simulink model "sampleModel2062_4"  (R2023a)
settings: Solver=VariableStepAuto  StartTime=0.0  StopTime=10.0  RelTol=1e-3
libraries: simulink x2
settings Model: Creator=user1  LastModifiedBy=user1

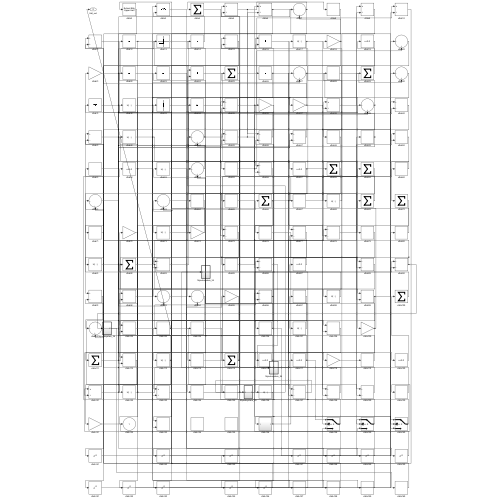
[thumbnail: Simulink's stored preview of the top-level diagram]
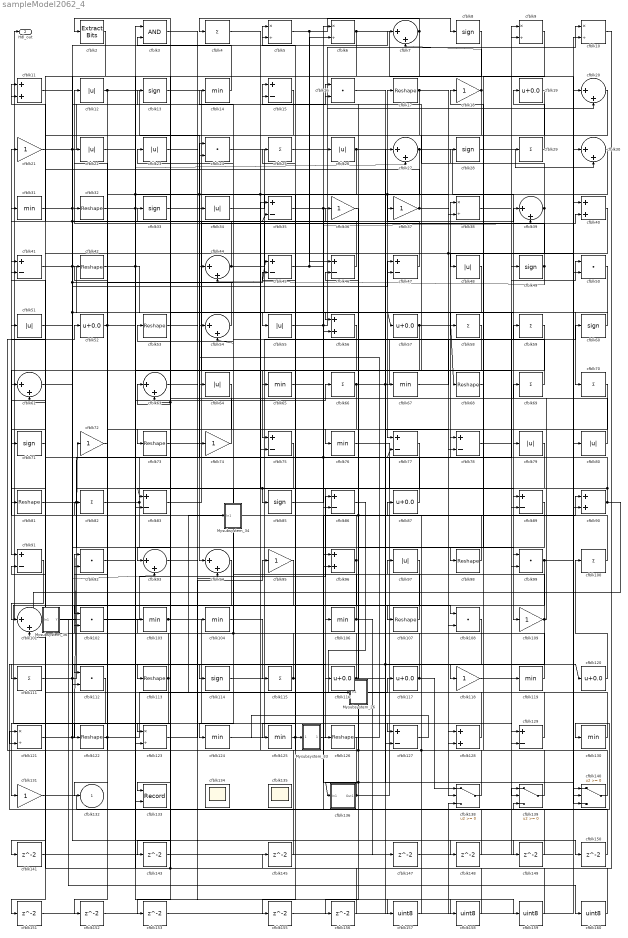
== system sampleModel2062_4 ==
  Mysubsystem_26 : Subsystem  TreatAsAtomicUnit=on  RTWFcnName=Mysubsystem_26
      settings: RTWFcnNameOpts=User specified  RTWFileNameOpts=Use function name
  Mysubsystem_33 : Subsystem  TreatAsAtomicUnit=on  RTWFcnName=Mysubsystem_33
      settings: RTWFcnNameOpts=User specified  RTWFileNameOpts=Use function name
  Mysubsystem_34 : Subsystem  TreatAsAtomicUnit=on  RTWFcnName=Mysubsystem_34
      settings: RTWFcnNameOpts=User specified  RTWFileNameOpts=Use function name
  Mysubsystem_36 : Subsystem  TreatAsAtomicUnit=on  RTWFcnName=Mysubsystem_36
      settings: RTWFcnNameOpts=User specified  RTWFileNameOpts=Use function name
  cfblk{5..6,9..10,38,121,123} (7 alike) : Product  Inputs=*/  OutDataTypeStr=uint8  RndMeth=Zero  SaturateOnIntegerOverflow=on
  cfblk{4,25,29,58..59,66,69..70,82,100,111,115} (12 alike) : Sum  Inputs=+  OutDataTypeStr=uint8
  cfblk{7,20,27,30,39,44,54,61,63,93..94,101} (12 alike) : Sum  Inputs=|++  OutDataTypeStr=uint8
  cfblk{16,24,50,92,99,102,108,112} (8 alike) : DotProduct  OutDataTypeStr=uint8
  cfblk{14,31,65,67,76,103..104,106,119,124..125,130} (12 alike) : MinMax  OutDataTypeStr=uint8
  cfblk{17,32,42,53,68,73,81,98,107,113,122,126} (12 alike) : Reshape
  cfblk{18,21,36..37,72,74,95,109,118,131} (10 alike) : Gain  OutDataTypeStr=uint8
  cfblk{11,40,56,90,96,128} (6 alike) : Sum  OutDataTypeStr=uint8
  cfblk{8,13,28,33,49,60,71,85,114} (9 alike) : Signum
  cfblk{19,52,57,87,116..117,120} (7 alike) : Bias  Bias=0.0  SaturateOnIntegerOverflow=off
  cfblk{12,22..23,26,34,48,51,55,64,79..80,97} (12 alike) : Abs  OutDataTypeStr=uint8  SaturateOnIntegerOverflow=off
  cfblk{15,35,41,45..47,75,77..78,83,86,89,91,127,129} (15 alike) : Sum  Inputs=+-  OutDataTypeStr=uint8
  cfblk133 : Record  FileSettingsInternal="{\"entries\":[{\"content\":{\"excelSettings\":{\"content\":{},\"type\":\"Streamout.ExcelSettings\"}},\"type\":\"Streamout.FileSettingStorage\",\"uuid\":\"\"}],\"packageUris\":[\"http:\\/\\/schema.mathworks.com\\/mf0\\/streamout_blocks\\/R2020a\"],\"version\":\"1.0\"}"  Layout=[1 1]  SignalsInternal="{\"entries\":[{\"content\":{\"signals\":[{\"content\":{\"blockPath\":[],\"dimensions\":[1],\"domain\":\"\",\"lineColor\":\"#a2142f\",\"plots\":[1],\"port\":1,\"signalID\":60930,\"signalName\":\"cfblk97\"},\"type\":\"RecordBlkView.Signal\",\"uuid\":\"\"},{\"content\":{\"blockPath\":[],\"dimensions\":[1],\"domain\":\"\",\"lineColor\":\"#139fff\",\"plots\":[1],\"port\":2,\"signalID\":60933,\"signalName\":\"cfblk30\"},\"type\":\"RecordBlkView.Signal\",\"uuid\":\"\"}]},\"type\":\"RecordBlkView.InputSignals\",\"uuid\":\"\"}],\"packageUris\":[\"http:\\/\\/schema.mathworks.com\\/mf0\\/streamout_blocks\\/R2020a\"],\"version\":\"1.0\"}"  VisualizationBindings="{\"xyplotplugin\":{\"info\":[{\"series\":[{\"bindingParametersList\":[{\"parameter\":\"X-Axis\",\"signalID\":60930,\"signalName\":\"cfblk97\"},{\"parameter\":\"Y-Axis\",\"signalID\":60933,\"signalName\":\"cfblk30\"}],\"seriesID\":23448}],\"subplotID\":1}]}}"  CompatibilityTag=XY  st=-1
  cfblk134 : Scope
      settings: Floating=on
  cfblk135 : Scope
      settings: Floating=on
  cfblk136 : Subsystem
      settings: LibrarySourceBlock=|
      | hdlsllib/Ports &
      | Subsystems/Subsystem
  cfblk138 : Switch  OutDataTypeStr=uint8  SaturateOnIntegerOverflow=off  InputSameDT=off
  cfblk139 : Switch  OutDataTypeStr=uint8  SaturateOnIntegerOverflow=off  InputSameDT=off
  cfblk140 : Switch  OutDataTypeStr=uint8  SaturateOnIntegerOverflow=off  InputSameDT=off
  cfblk{141,143,145,147..153,155..156} (12 alike) : Delay  SampleTime=1
  cfblk{157..160} (4 alike) : DataTypeConversion  OutDataTypeStr=uint8  SaturateOnIntegerOverflow=off  RndMeth=Floor
  cfblk2 : simulink/Logic and Bit Operations/Extract Bits  bitsToExtract=Upper half  numBits=8  bitIdxRange=[0 7]  outScalingMode=Preserve fixed-point scaling
      settings: LibrarySourceBlock=|
      | hdlsllib/Logic and Bit
      | Operations/Extract Bits
  cfblk3 : Logic  AllPortsSameDT=off  OutDataTypeStr=boolean
  cfblk132 : Outport  OutDataTypeStr=uint8  VectorParamsAs1DForOutWhenUnconnected=off
  Hdl_out : Outport  Port=2  OutDataTypeStr=uint8
  wires:
  cfblk30/1 -> cfblk34/1, cfblk133/2, cfblk75/2, cfblk77/1
  cfblk136/1(Out1) -> cfblk38/1, cfblk42/1
  cfblk29/1 -> cfblk19/1
  cfblk13/1 -> cfblk55/1
  cfblk47/1 -> cfblk17/1
  cfblk69/1 -> cfblk23/1
  cfblk56/1 -> cfblk91/1
  cfblk32/1 -> cfblk27/2, cfblk158/1
  cfblk120/1 -> cfblk100/1
  cfblk19/1 -> cfblk93/1, cfblk63/2
  cfblk12/1 -> cfblk94/1, cfblk132/1
  cfblk101/1 -> cfblk107/1
  cfblk27/1 -> cfblk109/1, cfblk155/1
  cfblk14/1 -> cfblk2/1
  cfblk90/1 -> Mysubsystem_36/1(In1), cfblk85/1, cfblk83/1, cfblk41/1
  cfblk71/1 -> cfblk127/1
  cfblk81/1 -> cfblk89/1, cfblk138/2
  cfblk121/1 -> cfblk35/2, cfblk7/1, cfblk45/1, cfblk72/1
  cfblk114/1 -> cfblk9/1
  cfblk126/1 -> cfblk52/1
  cfblk16/1 -> cfblk118/1
  cfblk98/1 -> cfblk21/1
  cfblk140/1 -> cfblk87/1, cfblk36/1
  cfblk109/1 -> cfblk14/1, cfblk69/1, cfblk123/2
  cfblk79/1 -> cfblk127/2
  cfblk52/1 -> cfblk122/1, cfblk159/1
  cfblk49/1 -> cfblk12/1, cfblk44/2
  cfblk51/1 -> cfblk57/1, cfblk47/1
  cfblk131/1 -> cfblk130/1
  cfblk41/1 -> cfblk139/2, cfblk93/2
  cfblk55/1 -> cfblk10/1, cfblk39/2
  cfblk96/1 -> cfblk32/1, cfblk114/1
  cfblk111/1 -> cfblk24/1, cfblk47/2
  cfblk50/1 -> cfblk70/1
  cfblk122/1 -> cfblk117/1, cfblk92/2
  cfblk77/1 -> cfblk126/1
  cfblk112/1 -> cfblk131/1
  cfblk42/1 -> cfblk56/1, cfblk65/1
  cfblk38/1 -> cfblk9/2
  cfblk130/1 -> cfblk61/1
  cfblk124/1 -> cfblk60/1
  cfblk5/1 -> cfblk8/1, cfblk46/1
  cfblk21/1 -> cfblk13/1, cfblk96/2
  cfblk57/1 -> cfblk68/1, cfblk75/1
  cfblk64/1 -> cfblk73/1
  cfblk102/1 -> cfblk86/1
  cfblk58/1 -> cfblk136/1(In1), cfblk156/1
  cfblk66/1 -> cfblk10/2, cfblk78/2, cfblk86/2
  cfblk125/1 -> cfblk15/1, cfblk90/1
  cfblk24/1 -> cfblk79/1
  cfblk91/1 -> cfblk101/1
  cfblk8/1 -> cfblk113/1
  cfblk104/1 -> cfblk115/1
  cfblk113/1 -> cfblk102/2, cfblk151/1
  cfblk73/1 -> cfblk40/2
  cfblk89/1 -> cfblk106/1
  cfblk15/1 -> cfblk101/2
  cfblk83/1 -> cfblk39/1
  cfblk80/1 -> cfblk31/1
  cfblk18/1 -> cfblk67/1, cfblk7/2
  cfblk76/1 -> cfblk119/1
  cfblk37/1 -> cfblk128/1, cfblk11/2
  cfblk103/1 -> cfblk128/2, Hdl_out/1
  cfblk74/1 -> cfblk33/1
  cfblk100/1 -> cfblk5/1, cfblk46/2
  cfblk68/1 -> cfblk18/1
  cfblk53/1 -> cfblk94/2
  cfblk92/1 -> cfblk66/1
  cfblk138/1 -> cfblk16/1, cfblk45/2
  cfblk106/1 -> cfblk44/1, cfblk147/1
  cfblk129/1 -> cfblk5/2
  cfblk118/1 -> cfblk129/1
  cfblk97/1 -> cfblk133/1
  cfblk35/1 -> cfblk20/2, cfblk140/2
  cfblk78/1 -> cfblk50/1
  cfblk119/1 -> cfblk103/1
  cfblk39/1 -> cfblk71/1, cfblk15/2
  cfblk4/1 -> cfblk89/2
  cfblk34/1 -> cfblk37/1
  cfblk54/1 -> cfblk22/1
  cfblk28/1 -> cfblk30/2
  cfblk59/1 -> cfblk64/1
  cfblk116/1 -> cfblk92/1, cfblk78/1
  cfblk26/1 -> cfblk120/1, cfblk140/3, cfblk112/1
  cfblk67/1 -> cfblk59/1
  cfblk46/1 -> cfblk24/2
  cfblk6/1 -> cfblk140/1, cfblk83/2
  cfblk20/1 -> cfblk98/1
  cfblk115/1 -> cfblk25/1, cfblk91/2
  cfblk75/1 -> cfblk124/1
  cfblk7/1 -> cfblk4/1, cfblk112/2
  cfblk61/1 -> cfblk99/1
  cfblk99/1 -> cfblk80/1, cfblk153/1
  cfblk139/1 -> cfblk28/1
  cfblk25/1 -> cfblk26/1
  cfblk87/1 -> cfblk61/2
  cfblk123/1 -> cfblk95/1
  cfblk36/1 -> cfblk76/1
  cfblk33/1 -> cfblk99/2
  cfblk60/1 -> cfblk58/1
  cfblk9/1 -> cfblk48/1
  cfblk82/1 -> cfblk104/1, cfblk49/1
  cfblk72/1 -> cfblk102/1
  cfblk108/1 -> cfblk121/2
  cfblk44/1 -> cfblk29/1, cfblk11/1
  cfblk22/1 -> cfblk38/2, cfblk108/2
  cfblk65/1 -> cfblk108/1
  cfblk40/1 -> cfblk125/1
  cfblk107/1 -> cfblk53/1
  cfblk23/1 -> cfblk74/1
  cfblk17/1 -> cfblk129/2, cfblk50/2, cfblk81/1
  cfblk117/1 -> cfblk54/2, cfblk82/1, cfblk138/1
  cfblk94/1 -> cfblk123/1
  cfblk45/1 -> cfblk56/2, cfblk6/2
  cfblk2/1 -> cfblk111/1
  cfblk31/1 -> cfblk116/1, cfblk16/2
  cfblk85/1 -> cfblk6/1, cfblk77/2
  cfblk95/1 -> cfblk141/1
  cfblk141/1 -> cfblk40/1
  cfblk48/1 -> cfblk143/1
  cfblk143/1 -> cfblk139/1
  cfblk10/1 -> cfblk145/1
  cfblk145/1 -> cfblk35/1
  cfblk147/1 -> cfblk30/1
  cfblk93/1 -> cfblk148/1
  cfblk148/1 -> cfblk96/1
  cfblk63/1 -> cfblk149/1
  cfblk149/1 -> cfblk139/3
  cfblk11/1 -> cfblk150/1
  cfblk150/1 -> cfblk121/1
  cfblk151/1 -> cfblk27/1
  cfblk70/1 -> cfblk152/1
  cfblk152/1 -> cfblk20/1
  cfblk153/1 -> cfblk138/3
  cfblk155/1 -> cfblk90/2
  cfblk156/1 -> cfblk41/2
  cfblk3/1 -> cfblk157/1
  cfblk157/1 -> cfblk97/1
  cfblk158/1 -> cfblk3/1
  cfblk159/1 -> cfblk3/2
  cfblk160/1 -> cfblk63/1, cfblk51/1
  cfblk86/1 -> Mysubsystem_26/1(In1)
  cfblk127/1 -> Mysubsystem_33/1(In1)
  Mysubsystem_33/1(Out1) -> cfblk54/1
  cfblk128/1 -> Mysubsystem_34/1(In1)
  Mysubsystem_36/1(Y) -> cfblk160/1

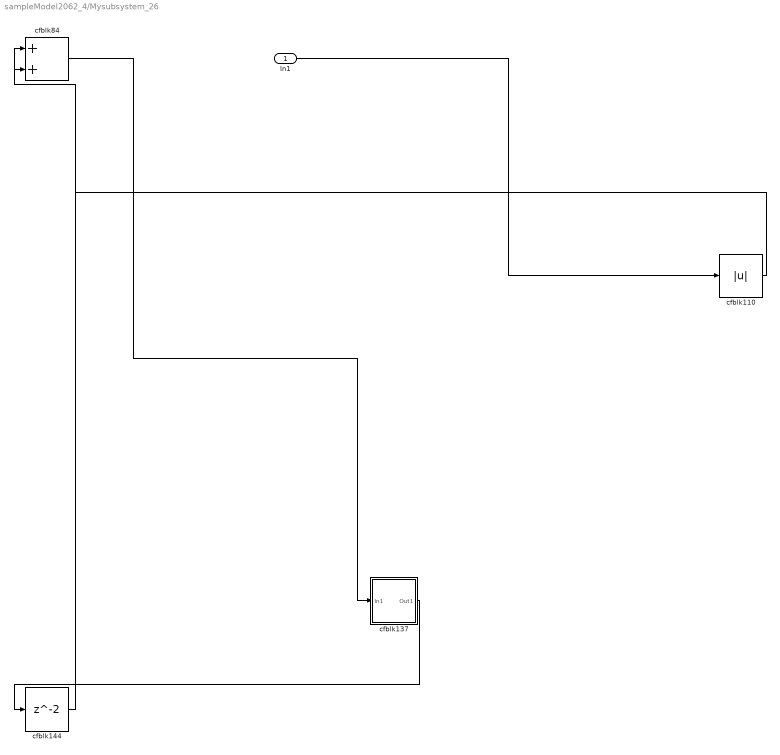
== system sampleModel2062_4/Mysubsystem_26 ==
  In1 : Inport
  cfblk110 : Abs  SaturateOnIntegerOverflow=off
  cfblk137 : Subsystem
      settings: LibrarySourceBlock=|
      | hdlsllib/Ports &
      | Subsystems/Subsystem
  cfblk144 : Delay  SampleTime=1
  cfblk84 : Sum
  wires:
  cfblk110/1 -> cfblk84/1
  cfblk84/1 -> cfblk137/1(In1)
  cfblk137/1(Out1) -> cfblk144/1
  In1/1 -> cfblk110/1
  cfblk144/1 -> cfblk84/2

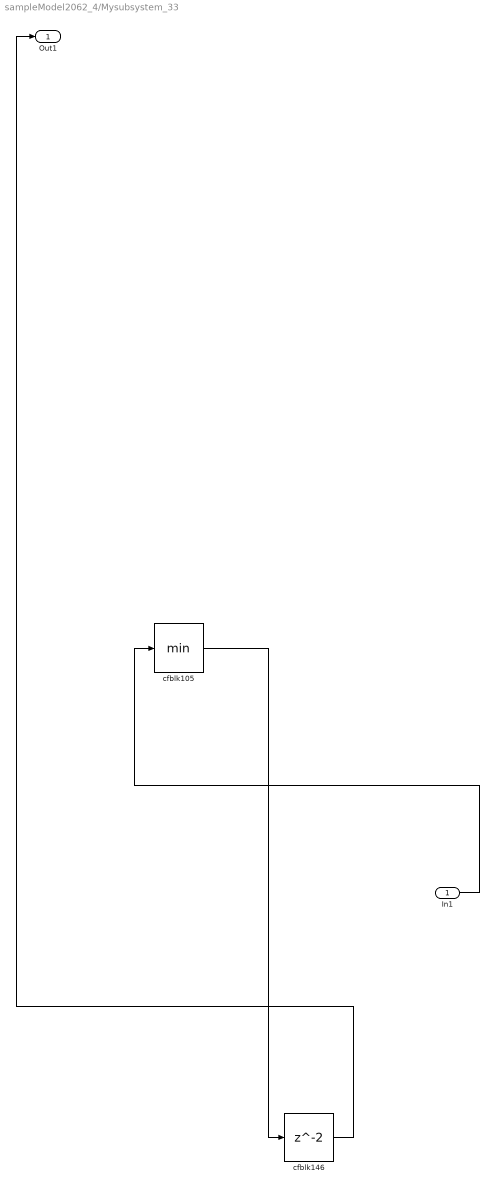
== system sampleModel2062_4/Mysubsystem_33 ==
  In1 : Inport
  cfblk105 : MinMax
  cfblk146 : Delay  SampleTime=1
  Out1 : Outport
  wires:
  cfblk105/1 -> cfblk146/1
  In1/1 -> cfblk105/1
  cfblk146/1 -> Out1/1

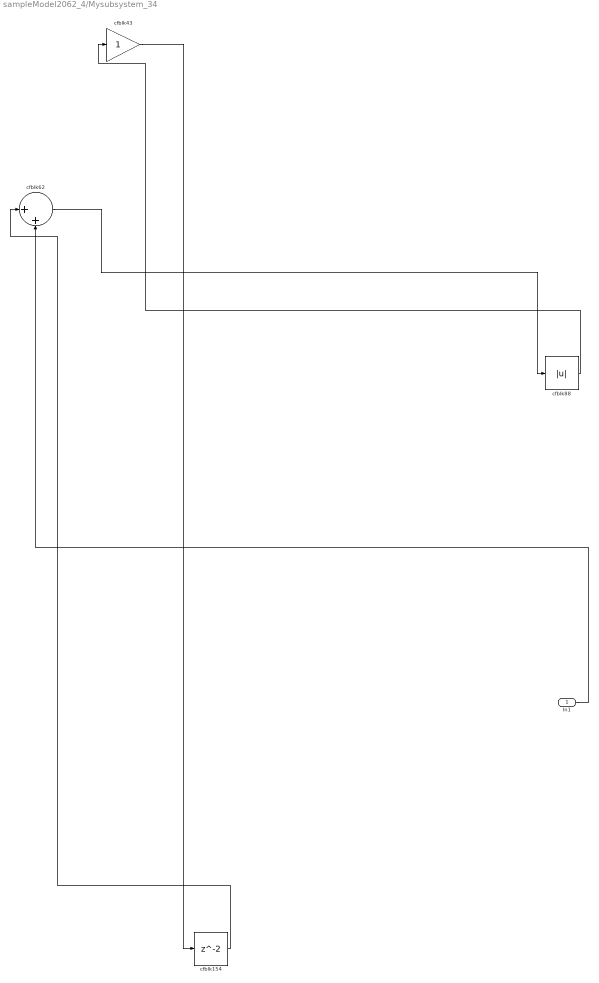
== system sampleModel2062_4/Mysubsystem_34 ==
  In1 : Inport
  cfblk154 : Delay  SampleTime=1
  cfblk43 : Gain
  cfblk62 : Sum  Inputs=|++
  cfblk88 : Abs  SaturateOnIntegerOverflow=off
  wires:
  cfblk88/1 -> cfblk43/1
  cfblk154/1 -> cfblk62/1
  cfblk62/1 -> cfblk88/1
  cfblk43/1 -> cfblk154/1
  In1/1 -> cfblk62/2

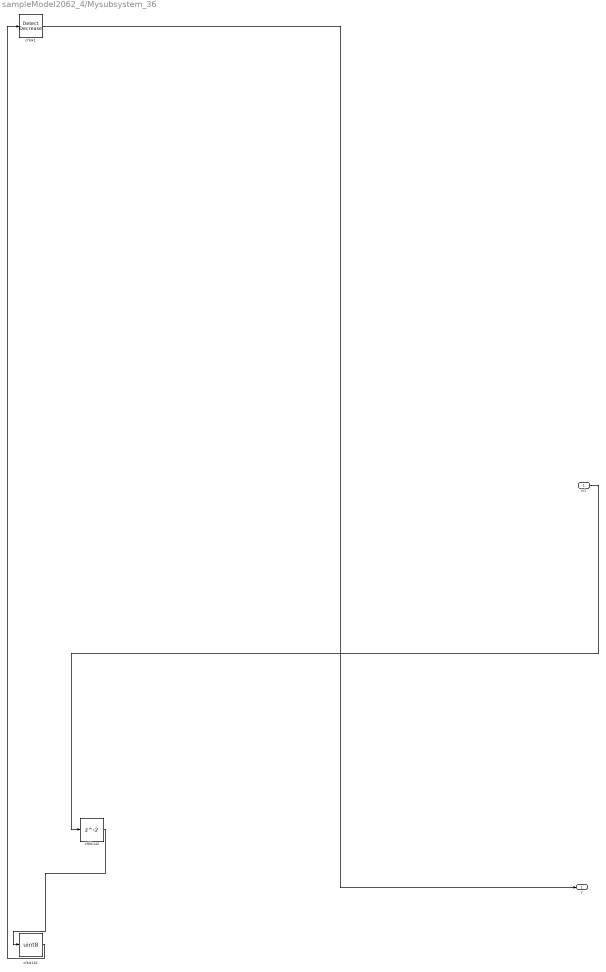
== system sampleModel2062_4/Mysubsystem_36 ==
  In1 : Inport
  cfblk1 : simulink/Logic and Bit Operations/Detect Decrease  vinit=0.0  OutDataTypeStr=boolean
      settings: LibrarySourceBlock=|
      | hdlsllib/Logic and Bit
      | Operations/Detect
      | Decrease
  cfblk142 : Delay  SampleTime=1
  cfblk161 : DataTypeConversion  OutDataTypeStr=uint8  SaturateOnIntegerOverflow=off  RndMeth=Floor
  Y : Outport
  wires:
  cfblk161/1 -> cfblk1/1
  cfblk142/1 -> cfblk161/1
  cfblk1/1 -> Y/1
  In1/1 -> cfblk142/1

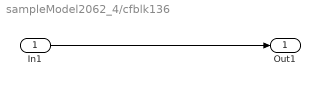
== system sampleModel2062_4/cfblk136 ==
  In1 : Inport
  Out1 : Outport
  wires:
  In1/1 -> Out1/1

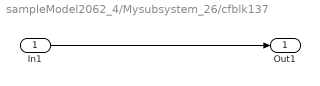
== system sampleModel2062_4/Mysubsystem_26/cfblk137 ==
  In1 : Inport
  Out1 : Outport
  wires:
  In1/1 -> Out1/1
